simulink model "RC1_Manual"  (R2017b)
settings: Solver=ode23t  StartTime=0.0  StopTime=5000  RelTol=1e-3  EnableMultiTasking=on
values from neighbouring files (symbols this model uses):
  Capacity = 31    [RC1_Manual.mat]    (also in dataInit.m; mayBeUsed.mat)
libraries: LiBatteryElements_lib x4, nesl_utility x4, fl_lib x3
settings Model: Creator=E540  LastModifiedBy=justs
settings DataIOCC: ExternalInput=[t,I_in]  MaxDataPoints=5000  LoadExternalInput=on  SaveFormat=Array  SaveTime=off  OutputTimes=[0,700]
settings OptimizationCC: LifeSpan=inf
settings DebuggingCC: SolverPrmCheckMsg=warning  SFUnexpectedBacktrackingDiag=warning  SFNoUnconditionalDefaultTransitionDiag=warning  SFExecutionAtInitializationDiag=none
settings HardwareCC: ProdBitPerPointer=32  ProdBitPerSizeT=32  ProdBitPerPtrDiffT=32  ProdLargestAtomicFloat=None  ProdIntDivRoundTo=Undefined  ProdEndianess=Unspecified  ProdWordSize=32  ProdHWDeviceType=32-bit Generic
settings ModelReferenceCC: PropagateSignalLabelsOutOfModel=off
settings CodeAppCC: StateflowObjectComments=on
settings GRTTargetCC: TargetLangStandard=C89/C90 (ANSI)  GeneratePreprocessorConditionals=Disable all
settings ConfigComp: CovMetricSettings=dw  CovHtmlReporting=on  CovSaveCumulativeToWorkspaceVar=on  CovSaveSingleToWorkspaceVar=on  CovExternalEMLEnable=off  CovSFcnEnable=off
settings SimscapeCC: SimscapeNormalizeSystem=off

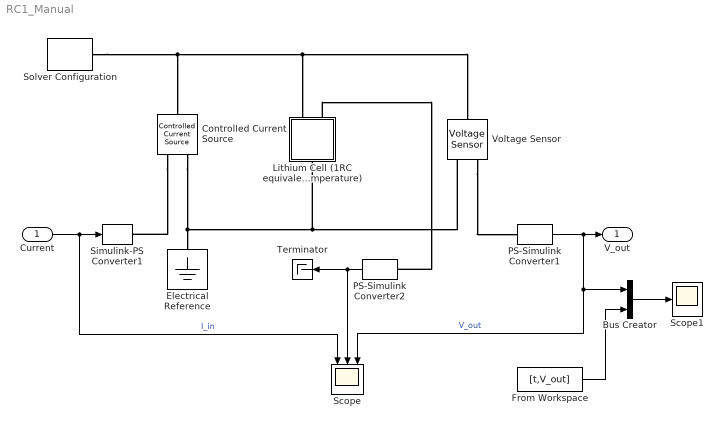
== system RC1_Manual ==
  Current : Inport
  Bus Creator : BusCreator  Inputs=2
  Controlled Current Source : fl_lib/Electrical/Electrical Sources/Controlled Current Source
  Electrical Reference : fl_lib/Electrical/Electrical Elements/Electrical Reference
  From Workspace : FromWorkspace  VariableName=[t,V_out]  SampleTime=0
  "Lithium Cell (1RC equivalent circuit model, single temperature)" : Subsystem
  PS-Simulink Converter1 : nesl_utility/PS-Simulink Converter  PhysicalDomain=network_engine_domain  SubClassName=ps_output  LeftPortType=input  RightPortType=output  PseudoPeriodic=off  Frequencies=[]  Unit=V  AffineConversion=off
  PS-Simulink Converter2 : nesl_utility/PS-Simulink Converter  PhysicalDomain=network_engine_domain  SubClassName=ps_output  LeftPortType=input  RightPortType=output  PseudoPeriodic=off  Frequencies=[]  Unit=1  AffineConversion=off
  Scope : Scope  NumInputPorts=3
  Scope1 : Scope
  Simulink-PS Converter1 : nesl_utility/Simulink-PS Converter  PhysicalDomain=network_engine_domain  SubClassName=ps_input  LeftPortType=input  RightPortType=output  PseudoPeriodic=off  Frequencies=[]  NoiseDistribution=none  NoiseParameters=[]  Unit=A  AffineConversion=off  FilteringAndDerivatives=zero  SimscapeFilterOrder=1  InputFilterTimeConstant=.001  UdotUserProvided=0
  Solver Configuration : nesl_utility/Solver Configuration  PhysicalDomain=network_engine_domain  SubClassName=solver  LeftPortType=input  RightPortType=generic  Accelerate=off  Tones=[]  Harmonics=[]  SimulateNoise=off  Profile=off  UseLocalSampling=off  EnableSwitchedLinearOptims=on  FrequencyDomain=off  UseCCode=off  RelTol=0.001  AbsTol=1e-06  MinStep=1e-09  ToWorkspace=off  RevertToSquareIcSolve=off  NumHomotopyIterations=100  PhasorMode=off  PhasorModeNumHarmonics=1  DoDC=off  ResidualTolerance=1e-09  UseLocalSolver=off  LocalSolverChoice=NE_BACKWARD_EULER_ADVANCER  LocalSolverSampleTime=0.001  DoFixedCost=off  MaxNonlinIter=3  MaxModeIter=2  LinearAlgebra=Sparse  DelaysMemoryBudget=1024  AutomaticFiltering=on  FilteringTimeConstant=0.001
  Terminator : Terminator
  Voltage Sensor : fl_lib/Electrical/Electrical Sensors/Voltage Sensor
  V_out : Outport
  wires:
  PS-Simulink Converter1/1 -> Bus Creator/1, Scope/3, V_out/1  "V_out"
  PS-Simulink Converter2/1 -> Terminator/1, Scope/2
  Current/1 -> Scope/1, Simulink-PS Converter1/1  "I_in"
  From Workspace/1 -> Bus Creator/2
  Bus Creator/1 -> Scope1/1
  connections:
  Solver Configuration/RConn1 -- Controlled Current Source/LConn1 -- "Lithium Cell (1RC equivalent circuit model, single temperature)"/LConn1 -- Voltage Sensor/LConn1
  Controlled Current Source/RConn1 -- Simulink-PS Converter1/RConn1
  Controlled Current Source/RConn2 -- Electrical Reference/LConn1 -- Voltage Sensor/RConn2 -- "Lithium Cell (1RC equivalent circuit model, single temperature)"/RConn1
  Voltage Sensor/RConn1 -- PS-Simulink Converter1/LConn1
  "Lithium Cell (1RC equivalent circuit model, single temperature)"/LConn2 -- PS-Simulink Converter2/LConn1

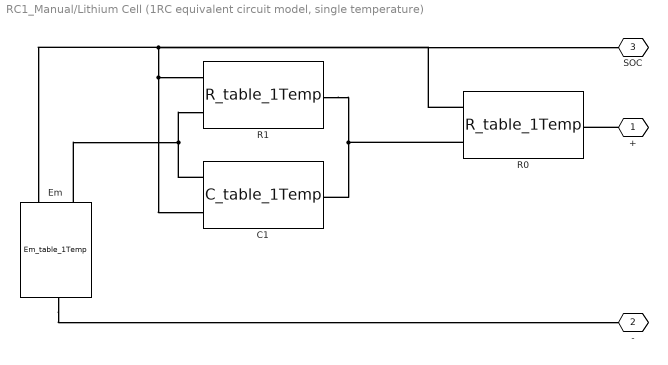
== system RC1_Manual/Lithium Cell (1RC equivalent circuit model, single temperature) ==
  C1 : LiBatteryElements_lib/C_table_1Temp  C_Table=C1 F  SOC_Table=SOC_LUT  v0=0 V
  Em : LiBatteryElements_lib/Em_table_1Temp  Em_Table=Em V  SOC_Table=SOC_LUT  C=Capacity hr*A  Qinit=Qe_init hr*A
  R0 : LiBatteryElements_lib/R_table_1Temp  R_Table=R0 Ohm  SOC_Table=SOC_LUT
  R1 : LiBatteryElements_lib/R_table_1Temp  R_Table=R1 Ohm  SOC_Table=SOC_LUT
  + : PMIOPort  Tag=PMCPort  Port=1  Side=Left
  - : PMIOPort  Tag=PMCPort  Port=2  Side=Right
  SOC : PMIOPort  Tag=PMCPort  Port=3  Side=Left
  connections:
  Em/LConn1 -- C1/LConn1 -- R1/LConn1
  +/RConn1 -- R0/RConn1
  Em/RConn1 -- -/RConn1
  R0/LConn2 -- SOC/RConn1 -- C1/LConn2 -- R1/LConn2 -- Em/LConn2
  R1/RConn1 -- R0/LConn1 -- C1/RConn1
